simulink model "generalSBandTransponder"  (R2021a)
settings: Solver=VariableStepAuto  StartTime=0.0  StopTime=500e-6  RelTol=1e-3
undefined symbols (not defined in the file): fdesignblkfcn, gcbh
libraries: dsparch4 x6, dspsrcs4 x5
settings Model: Creator=Zireael  LastModifiedBy=Zireael

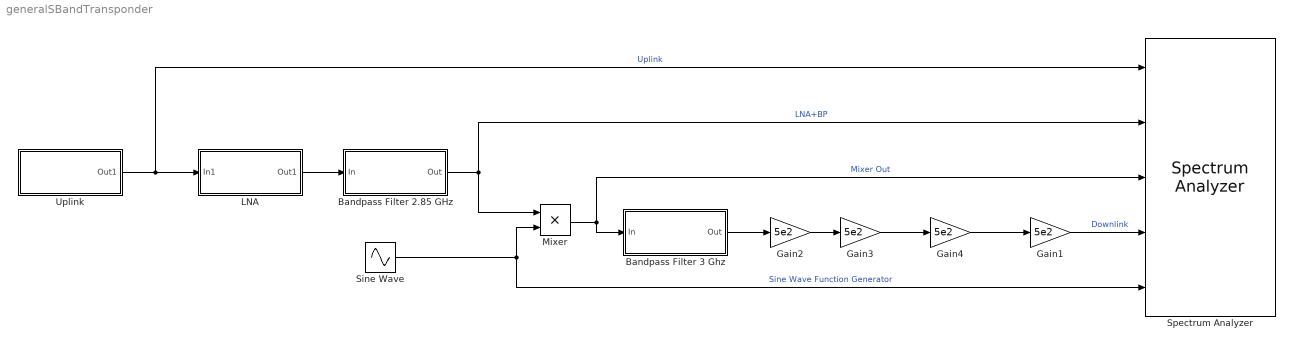
== system generalSBandTransponder ==
  Bandpass Filter 2.85 GHz : Subsystem  DialogController=fdesignblkfcn  InitFcn=fdesignblkfcn(gcbh, {'InitFcn'});  mask(Bandpass Filter){}
      mask help: Design a bandpass filter
      settings: CopyFcn=fdesignblkfcn(gcbh, {'CopyFcn'});
      mask Help: helpview(mapfilelocation('dsp'), 'dspbandpassfilter');
      mask Display: disp('Bandpass');
  Bandpass Filter 3 Ghz : Subsystem  DialogController=fdesignblkfcn  InitFcn=fdesignblkfcn(gcbh, {'InitFcn'});  mask(Bandpass Filter){}
      mask help: Design a bandpass filter
      settings: CopyFcn=fdesignblkfcn(gcbh, {'CopyFcn'});
      mask Help: helpview(mapfilelocation('dsp'), 'dspbandpassfilter');
      mask Display: disp('Bandpass');
  Gain{1..4} (4 alike) : Gain  Gain=5e2
  LNA : Subsystem
  Mixer : Product
  Sine Wave : Sin  Frequency=2*pi*3e9  SampleTime=1/(5e10)
  Spectrum Analyzer : SpectrumAnalyzer  NumInputPorts=5
  Uplink : Subsystem
  wires:
  Uplink/1(Out1) -> Spectrum Analyzer/1, LNA/1(In1)  "Uplink"
  LNA/1(Out1) -> Bandpass Filter 2.85 GHz/1(In)
  Bandpass Filter 2.85 GHz/1(Out) -> Spectrum Analyzer/2, Mixer/1  "LNA+BP"
  Mixer/1 -> Spectrum Analyzer/3, Bandpass Filter 3 Ghz/1(In)  "Mixer Out"
  Sine Wave/1 -> Spectrum Analyzer/5, Mixer/2  "Sine Wave Function Generator"
  Gain1/1 -> Spectrum Analyzer/4  "Downlink"
  Bandpass Filter 3 Ghz/1(Out) -> Gain2/1
  Gain2/1 -> Gain3/1
  Gain3/1 -> Gain4/1
  Gain4/1 -> Gain1/1

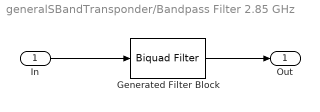
== system generalSBandTransponder/Bandpass Filter 2.85 GHz ==
  In : Inport
  Generated Filter Block : dsparch4/Biquad Filter  Tag=BlockMethodSubSystem  FilterSource=Dialog parameters  CoeffSource=Specify via dialog  FilterObject=BQF  IIRFiltStruct=Direct form II  BiQuadCoeffs=[0.100901896552980291 0 -0.100901896552980291 1 -1.88172643435111331 0.988795023202694301;0.0320481870649134831 0 -0.0320481870649134831 1 -1.81375996515562132 0.985922107596001185;0.0212714295186564664 0 -0.0212714295186564664 1 -1.85418994681885207 0.982797479845545219;0.0225484485824629828 0 -0.0225484485824629828 1 -1.83902440134983536 0.981905929182880777;0.148699230758427753 0 -0.148699230758427753 1 -1.8997953409114563 0.997638918645822992;0.0189519568975844641 0 -0.0189519568975844641 1 -1.8068507346376661 0.996750510733411255;0.0503528664753742777 0 -0.0503528664753742777 1 -1.86881465932585034 0.985242600028019777;0.0195784638130385401 0 -0.0195784638130385401 1 -1.82492534573115739 0.982912733075346989;0.138198153094904519 0 -0.138198153094904519 1 -1.89219086045647322 0.993035683047971185;1.61411555275832419 0 -1.61411555275832419 1 -1.80731224235916743 0.990714091662622698]  ScaleValues=[0.00362709459051515585;1;1;1;1;1;1;1;1;1;1]  IC=0  ICnum=0  ICden=0  a0Flag=Warning  optimizeScaleValues=off  ScaleValueMode=Specify via input port (g)  InputProcessing=Columns as channels (frame based)  roundingMode=Floor  overflowMode=off  scaleValueFracLength=14  denProdOutputFracLength=30  denAccumFracLength=30  secondMemoryFracLength=15
  Out : Outport  VectorParamsAs1DForOutWhenUnconnected=off
  wires:
  In/1 -> Generated Filter Block/1
  Generated Filter Block/1 -> Out/1

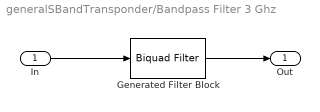
== system generalSBandTransponder/Bandpass Filter 3 Ghz ==
  In : Inport
  Generated Filter Block : dsparch4/Biquad Filter  Tag=BlockMethodSubSystem  FilterSource=Dialog parameters  CoeffSource=Specify via dialog  FilterObject=BQF  IIRFiltStruct=Direct form II  BiQuadCoeffs=[0.0375960179538544423 0 -0.0375960179538544423 1 -1.86820599454386116 0.995150844578175708;0.0123915552255431122 0 -0.0123915552255431122 1 -1.84143364658751207 0.994690754556567303;0.00835007898429048281 0 -0.00835007898429048281 1 -1.85649228446720627 0.992981351881712437;0.0110741395427019652 0 -0.0110741395427019652 1 -1.85054243093471782 0.992839254762510559;0.0533706048494430249 0 -0.0533706048494430249 1 -1.87644196645458639 0.998945700016637517;0.00751116051654214176 0 -0.00751116051654214176 1 -1.83940879437065252 0.998803168715563627;0.0187496227877654159 0 -0.0187496227877654159 1 -1.86256529732604115 0.993788866944457339;0.00947131662854122473 0 -0.00947131662854122473 1 -1.84532462006939224 0.993416801540596195;0.0501943576477351036 0 -0.0501943576477351036 1 -1.87295102879225572 0.996922883846880437;1.43988740320674879 0 -1.43988740320674879 1 -1.83936189010475681 0.996550322047287884]  ScaleValues=[0.00170258500224398685;1;1;1;1;1;1;1;1;1;1]  IC=0  ICnum=0  ICden=0  a0Flag=Warning  optimizeScaleValues=off  ScaleValueMode=Specify via input port (g)  InputProcessing=Columns as channels (frame based)  roundingMode=Floor  overflowMode=off  scaleValueFracLength=14  denProdOutputFracLength=30  denAccumFracLength=30  secondMemoryFracLength=15
  Out : Outport  VectorParamsAs1DForOutWhenUnconnected=off
  wires:
  In/1 -> Generated Filter Block/1
  Generated Filter Block/1 -> Out/1

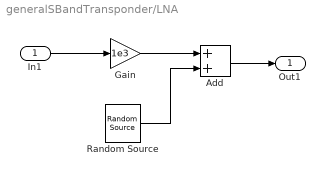
== system generalSBandTransponder/LNA ==
  In1 : Inport
  Add : Sum
  Gain : Gain  Gain=1e3
  Random Source : dspsrcs4/Random Source  SrcType=Gaussian  NormMethod=Ziggurat  CltLength=12  MinVal=0  MaxVal=1  MeanVal=0  VarVal=1e-3  RepMode=Not repeatable  rawSeed=1  IsInherit=off  SampMode=Discrete  SampTime=1/(5e10)  SampFrame=1  DataType=Double  OutComplex=Real  OutputFrames=off
  Out1 : Outport
  wires:
  Random Source/1 -> Add/2
  Gain/1 -> Add/1
  Add/1 -> Out1/1
  In1/1 -> Gain/1

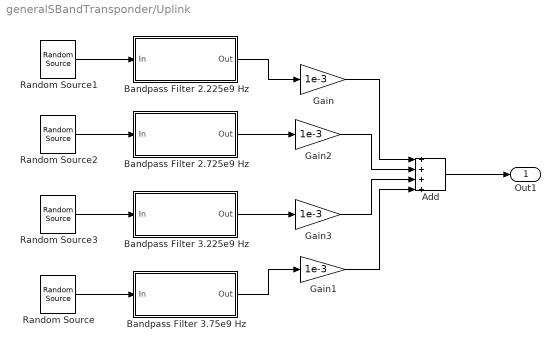
== system generalSBandTransponder/Uplink ==
  Add : Sum  Inputs=++++
  Bandpass Filter 2.225e9 Hz : Subsystem  DialogController=fdesignblkfcn  InitFcn=fdesignblkfcn(gcbh, {'InitFcn'});  mask(Bandpass Filter){}
      mask help: Design a bandpass filter
      settings: CopyFcn=fdesignblkfcn(gcbh, {'CopyFcn'});
      mask Help: helpview(mapfilelocation('dsp'), 'dspbandpassfilter');
      mask Display: disp('Bandpass');
  Bandpass Filter 2.725e9 Hz : Subsystem  DialogController=fdesignblkfcn  InitFcn=fdesignblkfcn(gcbh, {'InitFcn'});  mask(Bandpass Filter){}
      mask help: Design a bandpass filter
      settings: CopyFcn=fdesignblkfcn(gcbh, {'CopyFcn'});
      mask Help: helpview(mapfilelocation('dsp'), 'dspbandpassfilter');
      mask Display: disp('Bandpass');
  Bandpass Filter 3.225e9 Hz : Subsystem  DialogController=fdesignblkfcn  InitFcn=fdesignblkfcn(gcbh, {'InitFcn'});  mask(Bandpass Filter){}
      mask help: Design a bandpass filter
      settings: CopyFcn=fdesignblkfcn(gcbh, {'CopyFcn'});
      mask Help: helpview(mapfilelocation('dsp'), 'dspbandpassfilter');
      mask Display: disp('Bandpass');
  Bandpass Filter 3.75e9 Hz : Subsystem  DialogController=fdesignblkfcn  InitFcn=fdesignblkfcn(gcbh, {'InitFcn'});  mask(Bandpass Filter){}
      mask help: Design a bandpass filter
      settings: CopyFcn=fdesignblkfcn(gcbh, {'CopyFcn'});
      mask Help: helpview(mapfilelocation('dsp'), 'dspbandpassfilter');
      mask Display: disp('Bandpass');
  Gain{,1..3} (4 alike) : Gain  Gain=1e-3
  Random Source{,1..3} (4 alike) : dspsrcs4/Random Source  SrcType=Gaussian  NormMethod=Ziggurat  CltLength=12  MinVal=0  MaxVal=1  MeanVal=0  VarVal=1  RepMode=Not repeatable  rawSeed=1  IsInherit=off  SampMode=Discrete  SampTime=1/(5e10)  SampFrame=1  DataType=Double  OutComplex=Real  OutputFrames=off
  Out1 : Outport
  wires:
  Random Source1/1 -> Bandpass Filter 2.225e9 Hz/1(In)
  Random Source/1 -> Bandpass Filter 3.75e9 Hz/1(In)
  Bandpass Filter 2.225e9 Hz/1(Out) -> Gain/1
  Bandpass Filter 3.75e9 Hz/1(Out) -> Gain1/1
  Gain/1 -> Add/1
  Gain1/1 -> Add/4
  Add/1 -> Out1/1
  Bandpass Filter 2.725e9 Hz/1(Out) -> Gain2/1
  Random Source2/1 -> Bandpass Filter 2.725e9 Hz/1(In)
  Random Source3/1 -> Bandpass Filter 3.225e9 Hz/1(In)
  Bandpass Filter 3.225e9 Hz/1(Out) -> Gain3/1
  Gain3/1 -> Add/3
  Gain2/1 -> Add/2

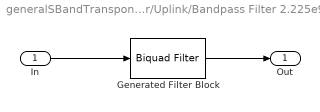
== system generalSBandTransponder/Uplink/Bandpass Filter 2.225e9 Hz ==
  In : Inport
  Generated Filter Block : dsparch4/Biquad Filter  Tag=BlockMethodSubSystem  FilterSource=Dialog parameters  CoeffSource=Specify via dialog  FilterObject=BQF  IIRFiltStruct=Direct form II  BiQuadCoeffs=[0.0537957550652699359 0 -0.0537957550652699359 1 -1.93311485321337417 0.997539426414004282;0.0184546650081867034 0 -0.0184546650081867034 1 -1.90558804798282955 0.997078229423412954;0.0156645592904149297 0 -0.0156645592904149297 1 -1.92131498005721646 0.994847498476399972;0.00915391213914710025 0 -0.00915391213914710025 1 -1.91463308186049797 0.994630503907973917;0.0275332491397737543 0 -0.0275332491397737543 1 -1.92779125558824993 0.995901233582924261;0.00511870674375507987 0 -0.00511870674375507987 1 -1.90897032946307332 0.99539433134329891;0.062383751668664153 0 -0.062383751668664153 1 -1.9366623080720875 0.999492294493084632;0.00507645013641344362 0 -0.00507645013641344362 1 -1.90538746276710835 0.999381499380513683;0.0457335278266697495 0 -0.0457335278266697495 1 -1.93064312987679632 0.996664468993969654;0.0208058773638621353 0 -0.0208058773638621353 1 -1.90692428026681604 0.996134678229191883;0.00674867764884718585 0 -0.00674867764884718585 1 -1.917927883173137 0.994621590217831697;0.0205767273813734497 0 -0.0205767273813734497 1 -1.92464591211570424 0.995284263013016091;0.0112119833077121978 0 -0.0112119833077121978 1 -1.91159214359028873 0.994887956654472827;0.0597059060778688117 0 -0.0597059060778688117 1 -1.93513863502750416 0.998492634797562228;1.98167149927535613 0 -1.98167149927535613 1 -1.90505925764287243 0.998179588953853392]  ScaleValues=[0.000619921497028901275;1;1;1;1;1;1;1;1;1;1;1;1;1;1;1]  IC=0  ICnum=0  ICden=0  a0Flag=Warning  optimizeScaleValues=off  ScaleValueMode=Specify via input port (g)  InputProcessing=Columns as channels (frame based)  roundingMode=Floor  overflowMode=off  scaleValueFracLength=14  denProdOutputFracLength=30  denAccumFracLength=30  secondMemoryFracLength=15
  Out : Outport  VectorParamsAs1DForOutWhenUnconnected=off
  wires:
  In/1 -> Generated Filter Block/1
  Generated Filter Block/1 -> Out/1

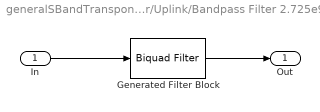
== system generalSBandTransponder/Uplink/Bandpass Filter 2.725e9 Hz ==
  In : Inport
  Generated Filter Block : dsparch4/Biquad Filter  Tag=BlockMethodSubSystem  FilterSource=Dialog parameters  CoeffSource=Specify via dialog  FilterObject=BQF  IIRFiltStruct=Direct form II  BiQuadCoeffs=[0.0528353767634784713 0 -0.0528353767634784713 1 -1.89761893618950328 0.997494475364245958;0.0185395627069431836 0 -0.0185395627069431836 1 -1.86430266764320818 0.997123161715483208;0.0153756171649529049 0 -0.0153756171649529049 1 -1.88363760816814896 0.994826243078679395;0.00931762420151795341 0 -0.00931762420151795341 1 -1.87558425836693798 0.99465175512353976;0.0270276293823802222 0 -0.0270276293823802222 1 -1.89136740244674906 0.995851682566848084;0.0050427958500742576 0 -0.0050427958500742576 1 -1.86865171522506901 0.995443859602757497;0.0614767243282268172 0 -0.0614767243282268172 1 -1.90160436583223613 0.999481515972048262;0.00537645854505560544 0 -0.00537645854505560544 1 -1.86359716393880315 0.999392276822959169;0.0450987031854676798 0 -0.0450987031854676798 1 -1.89473558080696325 0.996612757211635891;0.020461240735674905 0 -0.020461240735674905 1 -1.86607324393561647 0.996186365205189328;0.00686616171698697063 0 -0.00686616171698697063 1 -1.87956570852456784 0.994621590217831475;0.020228551159644264 0 -0.020228551159644264 1 -1.88762367516341856 0.995245474540472852;0.0117518867982447702 0 -0.0117518867982447702 1 -1.87188238473728985 0.994926731193197744;0.0580329156717120168 0 -0.0580329156717120168 1 -1.89993073688968872 0.99846215936405347;1.59674272612292212 0 -1.59674272612292212 1 -1.86345595576832435 0.998210055762638548]  ScaleValues=[0.000782477894518907686;1;1;1;1;1;1;1;1;1;1;1;1;1;1;1]  IC=0  ICnum=0  ICden=0  a0Flag=Warning  optimizeScaleValues=off  ScaleValueMode=Specify via input port (g)  InputProcessing=Columns as channels (frame based)  roundingMode=Floor  overflowMode=off  scaleValueFracLength=14  denProdOutputFracLength=30  denAccumFracLength=30  secondMemoryFracLength=15
  Out : Outport  VectorParamsAs1DForOutWhenUnconnected=off
  wires:
  In/1 -> Generated Filter Block/1
  Generated Filter Block/1 -> Out/1

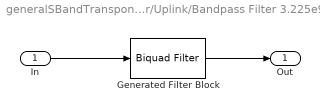
== system generalSBandTransponder/Uplink/Bandpass Filter 3.225e9 Hz ==
  In : Inport
  Generated Filter Block : dsparch4/Biquad Filter  Tag=BlockMethodSubSystem  FilterSource=Dialog parameters  CoeffSource=Specify via dialog  FilterObject=BQF  IIRFiltStruct=Direct form II  BiQuadCoeffs=[0.0521631377914760289 0 -0.0521631377914760289 1 -1.85464727495430104 0.997463042768485186;0.0185791132091203785 0 -0.0185791132091203785 1 -1.81564644560307897 0.997154583600724509;0.0152129114435178604 0 -0.0152129114435178604 1 -1.83853221957346991 0.994811422445887938;0.00944200916404356119 0 -0.00944200916404356119 1 -1.82912752029687953 0.99466657337761788;0.0266945893453514153 0 -0.0266945893453514153 1 -1.84749315600326525 0.995817090489240164;0.0047281674246837796 0 -0.0047281674246837796 1 -1.82094441662092921 0.995478438715301728;0.0605227509027845417 0 -0.0605227509027845417 1 -1.85904507594911728 0.999473971438812225;0.00592668283838243808 0 -0.00592668283838243808 1 -1.81444868247271351 0.999399820739521938;0.0446449341469691702 0 -0.0446449341469691702 1 -1.85136527089598557 0.996576626320735515;0.0202485977999102666 0 -0.0202485977999102666 1 -1.81784277416440432 0.99622248194716656;0.0069463011921669076 0 -0.0069463011921669076 1 -1.83378574671634453 0.994621590217831586;0.0199930151471045259 0 -0.0199930151471045259 1 -1.84316261264067505 0.995218415578003501;0.0119908461028401612 0 -0.0119908461028401612 1 -1.82477439859126545 0.994953782225068917;0.0574957070528425498 0 -0.0574957070528425498 1 -1.85723396868942281 0.998440835427185092;1.34349691417652006 0 -1.34349691417652006 1 -1.81448915600814575 0.998231374770693347]  ScaleValues=[0.000942061803180497702;1;1;1;1;1;1;1;1;1;1;1;1;1;1;1]  IC=0  ICnum=0  ICden=0  a0Flag=Warning  optimizeScaleValues=off  ScaleValueMode=Specify via input port (g)  InputProcessing=Columns as channels (frame based)  roundingMode=Floor  overflowMode=off  scaleValueFracLength=14  denProdOutputFracLength=30  denAccumFracLength=30  secondMemoryFracLength=15
  Out : Outport  VectorParamsAs1DForOutWhenUnconnected=off
  wires:
  In/1 -> Generated Filter Block/1
  Generated Filter Block/1 -> Out/1

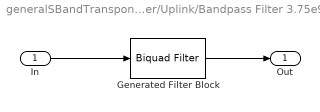
== system generalSBandTransponder/Uplink/Bandpass Filter 3.75e9 Hz ==
  In : Inport
  Generated Filter Block : dsparch4/Biquad Filter  Tag=BlockMethodSubSystem  FilterSource=Dialog parameters  CoeffSource=Specify via dialog  FilterObject=BQF  IIRFiltStruct=Direct form II  BiQuadCoeffs=[0.0576744214566959346 0 -0.0576744214566959346 1 -1.80380884826303833 0.997170738806604007;0.0206090312143415132 0 -0.0206090312143415132 1 -1.75399145205550688 0.996850213724905121;0.0169054941727511364 0 -0.0169054941727511364 1 -1.78360505802578917 0.994231069843514947;0.0105271518858667326 0 -0.0105271518858667326 1 -1.77160829955274779 0.99408059697874962;0.0295315617099678705 0 -0.0295315617099678705 1 -1.79491301499439238 0.99534128283812251;0.00510074802923406526 0 -0.00510074802923406526 1 -1.76103151584743856 0.994989447991702414;0.0668734813759797458 0 -0.0668734813759797458 1 -1.80909866064764024 0.999412961159968694;0.0068504644855992931 0 -0.0068504644855992931 1 -1.75206247072627885 0.999335891875659743;0.0493478592689018947 0 -0.0493478592689018947 1 -1.79974978286017917 0.99618445233697539;0.0224612157938098578 0 -0.0224612157938098578 1 -1.75695142643533231 0.995816491600662435;0.00773537972221244405 0 -0.00773537972221244405 1 -1.77756676424848692 0.994025401747606674;0.0221559729876706947 0 -0.0221559729876706947 1 -1.78946462560744579 0.994678889014715795;0.0134482367783744262 0 -0.0134482367783744262 1 -1.76600431380372314 0.994403970818751759;0.0634393311672077909 0 -0.0634393311672077909 1 -1.80695827496446859 0.998260438639945513;1.16364053780550147 0 -1.16364053780550147 1 -1.75232635839814166 0.998042760014084651]  ScaleValues=[0.00121490215335217223;1;1;1;1;1;1;1;1;1;1;1;1;1;1;1]  IC=0  ICnum=0  ICden=0  a0Flag=Warning  optimizeScaleValues=off  ScaleValueMode=Specify via input port (g)  InputProcessing=Columns as channels (frame based)  roundingMode=Floor  overflowMode=off  scaleValueFracLength=14  denProdOutputFracLength=30  denAccumFracLength=30  secondMemoryFracLength=15
  Out : Outport  VectorParamsAs1DForOutWhenUnconnected=off
  wires:
  In/1 -> Generated Filter Block/1
  Generated Filter Block/1 -> Out/1
